simulink model "Invert_Dynamic_Model"  (R2018a)
settings: Solver=VariableStepAuto  StartTime=0.0  StopTime=6  MaxStep=0.01  RelTol=1e-3  EnableMultiTasking=on
settings Model: Creator=ThanhUTC  LastModifiedBy=ShiningDanyang
settings OptimizationCC: LifeSpan=inf
settings DebuggingCC: SFUnexpectedBacktrackingDiag=warning  SFNoUnconditionalDefaultTransitionDiag=warning  SFExecutionAtInitializationDiag=none
settings CodeAppCC: StateflowObjectComments=on
settings GRTTargetCC: TargetLangStandard=C89/C90 (ANSI)  GeneratePreprocessorConditionals=Disable all
settings ConfigComp: CovMetricSettings=dw  CovHtmlReporting=on  CovSaveCumulativeToWorkspaceVar=on  CovSaveSingleToWorkspaceVar=on  CovExternalEMLEnable=off

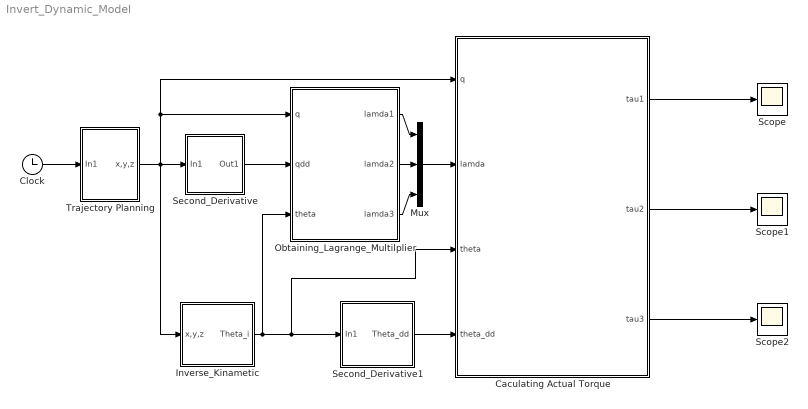
== system Invert_Dynamic_Model ==
  Caculating Actual Torque : MATLAB Function  TreatAsAtomicUnit=on
  Clock : Clock
  Inverse_Kinametic : Subsystem
  Mux : Mux  Inputs=3
  Obtaining_Lagrange_Multilplier : MATLAB Function  TreatAsAtomicUnit=on
  Scope : Scope
  Scope1 : Scope
  Scope2 : Scope
  Second_Derivative : Subsystem
  Second_Derivative1 : Subsystem
  Trajectory Planning : Subsystem
  wires:
  Clock/1 -> Trajectory Planning/1(In1)
  Trajectory Planning/1(x,y,z) -> Caculating Actual Torque/1(q), Obtaining_Lagrange_Multilplier/1(q), Inverse_Kinametic/1(x,y,z), Second_Derivative/1(In1)
  Second_Derivative/1(Out1) -> Obtaining_Lagrange_Multilplier/2(qdd)
  Inverse_Kinametic/1(Theta_i) -> Caculating Actual Torque/3(theta), Second_Derivative1/1(In1), Obtaining_Lagrange_Multilplier/3(theta)
  Second_Derivative1/1(Theta_dd) -> Caculating Actual Torque/4(theta_dd)
  Caculating Actual Torque/1(tau1) -> Scope/1
  Caculating Actual Torque/2(tau2) -> Scope1/1
  Caculating Actual Torque/3(tau3) -> Scope2/1
  Obtaining_Lagrange_Multilplier/2(lamda2) -> Mux/2
  Mux/1 -> Caculating Actual Torque/2(lamda)
  Obtaining_Lagrange_Multilplier/1(lamda1) -> Mux/1
  Obtaining_Lagrange_Multilplier/3(lamda3) -> Mux/3

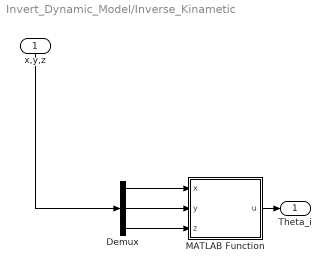
== system Invert_Dynamic_Model/Inverse_Kinametic ==
  x,y,z : Inport
  Demux : Demux  Outputs=3
  MATLAB Function : MATLAB Function  TreatAsAtomicUnit=on
  Theta_i : Outport
  wires:
  x,y,z/1 -> Demux/1
  MATLAB Function/1(u) -> Theta_i/1
  Demux/1 -> MATLAB Function/1(x)
  Demux/2 -> MATLAB Function/2(y)
  Demux/3 -> MATLAB Function/3(z)

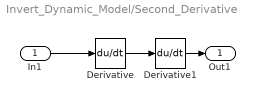
== system Invert_Dynamic_Model/Second_Derivative ==
  In1 : Inport
  Derivative : Derivative
  Derivative1 : Derivative
  Out1 : Outport
  wires:
  Derivative/1 -> Derivative1/1
  Derivative1/1 -> Out1/1
  In1/1 -> Derivative/1

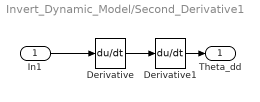
== system Invert_Dynamic_Model/Second_Derivative1 ==
  In1 : Inport
  Derivative : Derivative
  Derivative1 : Derivative
  Theta_dd : Outport
  wires:
  In1/1 -> Derivative/1
  Derivative1/1 -> Theta_dd/1
  Derivative/1 -> Derivative1/1

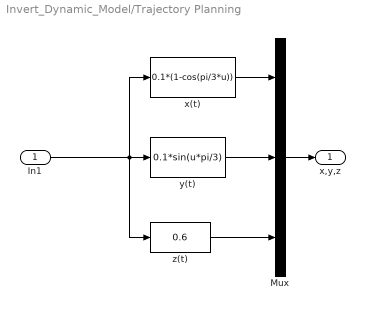
== system Invert_Dynamic_Model/Trajectory Planning ==
  In1 : Inport
  Mux : Mux  Inputs=3
  x(t) : Fcn  Expr=0.1*(1-cos(pi/3*u))
  y(t) : Fcn  Expr=0.1*sin(u*pi/3)
  z(t) : Fcn  Expr=0.6
  x,y,z : Outport
  wires:
  x(t)/1 -> Mux/1
  In1/1 -> z(t)/1, y(t)/1, x(t)/1
  y(t)/1 -> Mux/2
  z(t)/1 -> Mux/3
  Mux/1 -> x,y,z/1

== matlab function Invert_Dynamic_Model/Obtaining_Lagrange_Multilplier ==
  data: q input; lamda1 output; qdd input; theta input; lamda2 output; lamda3 output
function [lamda1, lamda2, lamda3] = fcn(q,qdd,theta)
%#codegen
% Phuong trinh vi phan cua ban may viet dc o dang
% A*lamda = B
% Trong do lamda = [lamda1; lamda2; lamda3]
% va A , B la cac ma tran
l1 = 0.3; l2 = 0.4; 
r = 0.06-0.2;
phi1 = 1.5708; phi2 = 3.6652; phi3 = 5.7596;
mo = 0.712; mp = 0.3; m2 = 2*0.452; m1 = 0.456;
g = 9.8;
%-------------------------------------------
x = q(1); y = q(2); z = q(3);
xdd = qdd(1); ydd = qdd(2); zdd = qdd(3);
theta1 = theta(1); theta2 = theta(2); theta3 = theta(3);
% Xay dung ma tran A
%hang 1
A11 = x+r*cos(phi1)-l1*cos(theta1)*cos(phi1);
A12 = x+r*cos(phi2)-l1*cos(theta2)*cos(phi2);
A13 = x+r*cos(phi3)-l1*cos(theta3)*cos(phi3);
%hang 2
A21 = y + r*sin(phi1)-l1*cos(theta1)*sin(phi1);
A22 = y + r*sin(phi2)-l1*cos(theta2)*sin(phi2);
A23 = y + r*sin(phi3)-l1*cos(theta3)*sin(phi3);
%hang 3
A31 = z - l1*sin(theta1);
A32 = z - l1*sin(theta2);
A33 = z - l1*sin(theta3);
A = [A11 A12 A13; A21 A22 A23; A31 A32 A33];
% Xay dung ma tran B
B11 = 0.5*(mo+mp+3*m2)*xdd;
B21 = 0.5*(mo+mp+3*m2)*ydd;
B31 = 0.5*(mo+mp+3*m2)*zdd + (mo+mp+3*m2)*g;
B = [B11;B21;B31];
lamda = inv(A)*B;   % Giai he phuong trinh de tim nhan tu lagrange lamda 
lamda1 = lamda(1);
lamda2 = lamda(2);
lamda3 = lamda(3);

== matlab function Invert_Dynamic_Model/Inverse_Kinametic/MATLAB Function ==
  data: x input; u output; y input; z input
function u = fcn(x,y,z)
%Tinhs cacs bieeur thucws a,b, c
l1 = 0.3; l2 = 0.4; 
phi = [1.5708;3.6652;5.7596];
r = 0.06-0.2;
a = 2*l1*(r-x*cos(phi)-y*sin(phi));
b = 2*z*l1;
c = x^2 + y^2 + z^2 +r^2 +l1^2 -l2^2 +2*r*(x*cos(phi)-y*sin(phi));
anfa = asin (a/(sqrt(a.^2+b.^2)));
theta1 = asin (c/(sqrt(a.^2+b.^2)))-anfa;
theta2 = pi - asin(c/(sqrt(a.^2+b.^2)))+anfa;
theta = [0;0;0];
for i=1:3
    if (theta1(i)>= -0.925)&&(theta1(i) <= 2) % Gioi han cua khau chu dong
        theta(i)=theta1(i);
    end 
    if (theta2(i)>= -0.925)&&(theta2(i) <= 2) % Gioi han cua khau chu dong
        theta(i)=theta2(i);
    end 
end
u = theta;
%#codegen

== matlab function Invert_Dynamic_Model/Caculating Actual Torque ==
  data: q input; lamda input; theta input; tau1 output; theta_dd input; tau2 output; tau3 output
function [tau1, tau2, tau3] = fcn(q, lamda,theta, theta_dd)
%#codegen
l1 = 0.3; l2 = 0.4; 
r = 0.06-0.2;
phi1 = 1.5708; phi2 = 3.6652; phi3 = 5.7596;
r = -0.15;
mo = 0.712; mp = 0.3; m2 = 2*0.452; m1 = 0.456
g = 9.8;
%------------------------------
x = q(1); y = q(2); z = q(3);
theta1 = theta(1); theta2 = theta(2); theta3 = theta(3);
lamda1 = lamda(1); lamda2 = lamda(2); lamda3 = lamda(3);
theta1_dd = theta_dd(1); theta2_dd = theta_dd(2); theta3_dd = theta_dd(3);
%tinh cac momen
tau1 = (1/3*m1+m2 )*l1^2*theta1_dd-2*lamda1*l1*((x*cos(phi1)+y*sin(phi1)+r)*sin(theta1)-z*cos(theta1));
tau2 = (1/3*m1+m2 )*l1^2*theta2_dd-2*lamda2*l1*((x*cos(phi2)+y*sin(phi2)+r)*sin(theta2)-z*cos(theta2));
tau3 = (1/3*m1+m2 )*l1^2*theta3_dd-2*lamda3*l1*((x*cos(phi3)+y*sin(phi3)+r)*sin(theta3)-z*cos(theta3));
%y = [tau1; tau2; tau3];
